simulink model "Quadcopter_ControllerWithNavigation"  (R2023b)
settings: Solver=FixedStepAuto  StartTime=0.0  StopTime=inf  RelTol=1e-3  EnableMultiTasking=on
undefined symbols (not defined in the file): dev, Main, pwm_output0, SampleTime
libraries: slpidlib x10, px4uORBlib x7, simulink x4, px4lib x3, uavalgslib x3, simulink_extras x1, sharedutil x1, sharedtransform x1
(part 2 of 3)

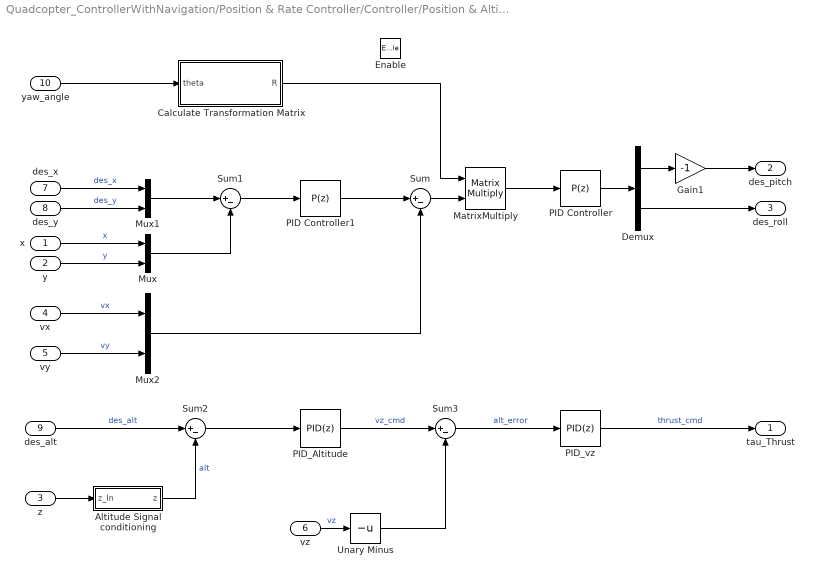
== system Quadcopter_ControllerWithNavigation/Position & Rate Controller/Controller/Position & Altitude controller ==
  x : Inport
  y : Inport  Port=2
  z : Inport  Port=3
  vx : Inport  Port=4
  vy : Inport  Port=5
  vz : Inport  Port=6
  des_x : Inport  Port=7
  des_y : Inport  Port=8
  des_alt : Inport  Port=9
  yaw_angle : Inport  Port=10
  Enable : EnablePort
  Altitude Signal conditioning : Subsystem
  Calculate Transformation Matrix : Subsystem
  Demux : Demux  Outputs=2
  Gain1 : Gain  Gain=-1
  MatrixMultiply : Product  Multiplication=Matrix(*)
  Mux : Mux  Inputs=2
  Mux1 : Mux  Inputs=2
  Mux2 : Mux  Inputs=2
  PID Controller : slpidlib/PID Controller  Controller=P  Form=Parallel  TimeDomain=Discrete-time  UseExternalTs=off  SampleTime=-1  IntegratorMethod=Forward Euler  FilterMethod=Forward Euler  ControllerParametersSource=internal  P=0.3  I=0  UseKiTs=off  D=0  N=20  UseFilter=on  TunerSelectOption=Transfer Function Based (PID Tuner App)  InitialConditionSource=internal  InitialConditionForIntegrator=0  InitialConditionForFilter=0  DifferentiatorICPrevScaledInput=0  ExternalReset=none  TrackingMode=off  Kt=1  LimitOutput=on  SatLimitsSource=internal  UpperSaturationLimit=20*pi/180  LowerSaturationLimit=-20*pi/180  LinearizeAsGain=on  AntiWindupMode=clamping  Kb=1  LimitIntegrator=off  UpperIntegratorSaturationLimit=inf  LowerIntegratorSaturationLimit=-inf  POutMin=[]  POutMax=[]  IOutMin=[]  IOutMax=[]  DOutMin=[]  DOutMax=[]  NOutMin=[]  NOutMax=[]  SumOutMin=[]  SumOutMax=[]  SaturationOutMin=[]  SaturationOutMax=[]  PParamMin=[]  PParamMax=[]  IParamMin=[]  IParamMax=[]  DParamMin=[]  DParamMax=[]  NParamMin=[]  NParamMax=[]  KbParamMin=[]  KbParamMax=[]  KtParamMin=[]  KtParamMax=[]  KbOutMin=[]  KbOutMax=[]  KtOutMin=[]  KtOutMax=[]  IntegratorOutMin=[]  IntegratorOutMax=[]  FilterOutMin=[]  FilterOutMax=[]  SumI1OutMin=[]  SumI1OutMax=[]  SumI2OutMin=[]  SumI2OutMax=[]  SumI3OutMin=[]  SumI3OutMax=[]  SumI4OutMin=[]  SumI4OutMax=[]  SumDOutMin=[]  SumDOutMax=[]  DifferentiatorOutMin=[]  DifferentiatorOutMax=[]  FilterDiffOutCoefMin=[]  FilterDiffOutCoefMax=[]  ReciprocalOutMin=[]  ReciprocalOutMax=[]  SumDenOutMin=[]  SumDenOutMax=[]  SumNumOutMin=[]  SumNumOutMax=[]  DivideOutMin=[]  DivideOutMax=[]  UdiffTsProdOutMin=[]  UdiffTsProdOutMax=[]  NTsProdOutMin=[]  NTsProdOutMax=[]  UintegralTsProdOutMin=[]  UintegralTsProdOutMax=[]  UngainTsProdOutMin=[]  UngainTsProdOutMax=[]  ClampingZeroOutDataTypeStr=Inherit: Inherit via back propagation  ClampingZeroOutMin=[]  ClampingZeroOutMax=[]  FilterDenConstantOutDataTypeStr=Inherit: Inherit via back propagation  FilterDenConstantOutMin=[]  FilterDenConstantOutMax=[]  PCopyOutDataTypeStr=Inherit: Inherit via back propagation  PCopyOutMin=[]  PCopyOutMax=[]  NCopyOutDataTypeStr=Inherit: Inherit via back propagation  NCopyOutMin=[]  NCopyOutMax=[]  IntegratorContinuousStateAttributes=''  IntegratorStateMustResolveToSignalObject=off  IntegratorRTWStateStorageClass=Auto  FilterContinuousStateAttributes=''  FilterStateMustResolveToSignalObject=off  FilterRTWStateStorageClass=Auto  ParallelPVariant=InternalParameters  IdealPVariant=Disabled  IVariant=Disabled  DVariant=Disabled  IntegratorVariant=Disabled  SatVariant=Enabled  AWVariant=Disabled  PCopyVariant=Disabled  TRVariant=Disabled  FdbkBlocksVariant=Forward  IdealPFdbkVariant=Disabled  SatFdbkVariant=Disabled  DerivativeFilterVariant=Disabled  NVariant=Disabled  NCopyVariant=Disabled_SignalSpec  FilterICVariant=Disabled  IntegratorICVariant=Disabled  ExternalResetVariant=Disabled  TRSumVariant=Passthrough  SumFdbkVariant=Disabled  SumVariant=Passthrough_P  TsampFilterVariant=InternalTs  TsampNgainVariant=Passthrough  TsampIntegralVariant=Disabled_SignalSpec  ExternalSaturationOutDataTypeStr=Inherit: Same as second input
  PID Controller1 : slpidlib/PID Controller  Controller=P  Form=Parallel  TimeDomain=Discrete-time  UseExternalTs=off  SampleTime=-1  IntegratorMethod=Forward Euler  FilterMethod=Forward Euler  ControllerParametersSource=internal  P=0.6  I=0  UseKiTs=off  D=0  N=20  UseFilter=on  TunerSelectOption=Transfer Function Based (PID Tuner App)  InitialConditionSource=internal  InitialConditionForIntegrator=0  InitialConditionForFilter=0  DifferentiatorICPrevScaledInput=0  ExternalReset=none  TrackingMode=off  Kt=1  LimitOutput=on  SatLimitsSource=internal  UpperSaturationLimit=4  LowerSaturationLimit=-4  LinearizeAsGain=on  AntiWindupMode=clamping  Kb=1  LimitIntegrator=off  UpperIntegratorSaturationLimit=inf  LowerIntegratorSaturationLimit=-inf  POutMin=[]  POutMax=[]  IOutMin=[]  IOutMax=[]  DOutMin=[]  DOutMax=[]  NOutMin=[]  NOutMax=[]  SumOutMin=[]  SumOutMax=[]  SaturationOutMin=[]  SaturationOutMax=[]  PParamMin=[]  PParamMax=[]  IParamMin=[]  IParamMax=[]  DParamMin=[]  DParamMax=[]  NParamMin=[]  NParamMax=[]  KbParamMin=[]  KbParamMax=[]  KtParamMin=[]  KtParamMax=[]  KbOutMin=[]  KbOutMax=[]  KtOutMin=[]  KtOutMax=[]  IntegratorOutMin=[]  IntegratorOutMax=[]  FilterOutMin=[]  FilterOutMax=[]  SumI1OutMin=[]  SumI1OutMax=[]  SumI2OutMin=[]  SumI2OutMax=[]  SumI3OutMin=[]  SumI3OutMax=[]  SumI4OutMin=[]  SumI4OutMax=[]  SumDOutMin=[]  SumDOutMax=[]  DifferentiatorOutMin=[]  DifferentiatorOutMax=[]  FilterDiffOutCoefMin=[]  FilterDiffOutCoefMax=[]  ReciprocalOutMin=[]  ReciprocalOutMax=[]  SumDenOutMin=[]  SumDenOutMax=[]  SumNumOutMin=[]  SumNumOutMax=[]  DivideOutMin=[]  DivideOutMax=[]  UdiffTsProdOutMin=[]  UdiffTsProdOutMax=[]  NTsProdOutMin=[]  NTsProdOutMax=[]  UintegralTsProdOutMin=[]  UintegralTsProdOutMax=[]  UngainTsProdOutMin=[]  UngainTsProdOutMax=[]  ClampingZeroOutDataTypeStr=Inherit: Inherit via back propagation  ClampingZeroOutMin=[]  ClampingZeroOutMax=[]  FilterDenConstantOutDataTypeStr=Inherit: Inherit via back propagation  FilterDenConstantOutMin=[]  FilterDenConstantOutMax=[]  PCopyOutDataTypeStr=Inherit: Inherit via back propagation  PCopyOutMin=[]  PCopyOutMax=[]  NCopyOutDataTypeStr=Inherit: Inherit via back propagation  NCopyOutMin=[]  NCopyOutMax=[]  IntegratorContinuousStateAttributes=''  IntegratorStateMustResolveToSignalObject=off  IntegratorRTWStateStorageClass=Auto  FilterContinuousStateAttributes=''  FilterStateMustResolveToSignalObject=off  FilterRTWStateStorageClass=Auto  ParallelPVariant=InternalParameters  IdealPVariant=Disabled  IVariant=Disabled  DVariant=Disabled  IntegratorVariant=Disabled  SatVariant=Enabled  AWVariant=Disabled  PCopyVariant=Disabled  TRVariant=Disabled  FdbkBlocksVariant=Forward  IdealPFdbkVariant=Disabled  SatFdbkVariant=Disabled  DerivativeFilterVariant=Disabled  NVariant=Disabled  NCopyVariant=Disabled_SignalSpec  FilterICVariant=Disabled  IntegratorICVariant=Disabled  ExternalResetVariant=Disabled  TRSumVariant=Passthrough  SumFdbkVariant=Disabled  SumVariant=Passthrough_P  TsampFilterVariant=InternalTs  TsampNgainVariant=Passthrough  TsampIntegralVariant=Disabled_SignalSpec  ExternalSaturationOutDataTypeStr=Inherit: Same as second input
  PID_Altitude : slpidlib/PID Controller  Controller=PID  Form=Parallel  TimeDomain=Discrete-time  UseExternalTs=off  SampleTime=-1  IntegratorMethod=Backward Euler  FilterMethod=Forward Euler  ControllerParametersSource=internal  P=1.5  I=0.01  UseKiTs=off  D=0.01  N=10  UseFilter=on  TunerSelectOption=Transfer Function Based (PID Tuner App)  InitialConditionSource=internal  InitialConditionForIntegrator=0  InitialConditionForFilter=0  DifferentiatorICPrevScaledInput=0  ExternalReset=none  TrackingMode=off  Kt=1  LimitOutput=on  SatLimitsSource=internal  UpperSaturationLimit=2  LowerSaturationLimit=-2  LinearizeAsGain=off  AntiWindupMode=clamping  Kb=1  LimitIntegrator=off  UpperIntegratorSaturationLimit=inf  LowerIntegratorSaturationLimit=-inf  POutMin=[]  POutMax=[]  IOutMin=[]  IOutMax=[]  DOutMin=[]  DOutMax=[]  NOutMin=[]  NOutMax=[]  SumOutMin=[]  SumOutMax=[]  SaturationOutMin=[]  SaturationOutMax=[]  PParamMin=[]  PParamMax=[]  IParamMin=[]  IParamMax=[]  DParamMin=[]  DParamMax=[]  NParamMin=[]  NParamMax=[]  KbParamMin=[]  KbParamMax=[]  KtParamMin=[]  KtParamMax=[]  KbOutMin=[]  KbOutMax=[]  KtOutMin=[]  KtOutMax=[]  IntegratorOutMin=[]  IntegratorOutMax=[]  FilterOutMin=[]  FilterOutMax=[]  SumI1OutMin=[]  SumI1OutMax=[]  SumI2OutMin=[]  SumI2OutMax=[]  SumI3OutMin=[]  SumI3OutMax=[]  SumI4OutMin=[]  SumI4OutMax=[]  SumDOutMin=[]  SumDOutMax=[]  DifferentiatorOutMin=[]  DifferentiatorOutMax=[]  FilterDiffOutCoefMin=[]  FilterDiffOutCoefMax=[]  ReciprocalOutMin=[]  ReciprocalOutMax=[]  SumDenOutMin=[]  SumDenOutMax=[]  SumNumOutMin=[]  SumNumOutMax=[]  DivideOutMin=[]  DivideOutMax=[]  UdiffTsProdOutMin=[]  UdiffTsProdOutMax=[]  NTsProdOutMin=[]  NTsProdOutMax=[]  UintegralTsProdOutMin=[]  UintegralTsProdOutMax=[]  UngainTsProdOutMin=[]  UngainTsProdOutMax=[]  ClampingZeroOutDataTypeStr=Inherit: Inherit via back propagation  ClampingZeroOutMin=[]  ClampingZeroOutMax=[]  FilterDenConstantOutDataTypeStr=Inherit: Inherit via back propagation  FilterDenConstantOutMin=[]  FilterDenConstantOutMax=[]  PCopyOutDataTypeStr=Inherit: Inherit via back propagation  PCopyOutMin=[]  PCopyOutMax=[]  NCopyOutDataTypeStr=Inherit: Inherit via back propagation  NCopyOutMin=[]  NCopyOutMax=[]  IntegratorContinuousStateAttributes=''  IntegratorStateMustResolveToSignalObject=off  IntegratorRTWStateStorageClass=Auto  FilterContinuousStateAttributes=''  FilterStateMustResolveToSignalObject=off  FilterRTWStateStorageClass=Auto  ParallelPVariant=InternalParameters  IdealPVariant=Disabled  IVariant=InternalParameters  DVariant=InternalParameters  IntegratorVariant=Discrete  SatVariant=Enabled  AWVariant=DiscClampingParallel  PCopyVariant=Disabled  TRVariant=Disabled  FdbkBlocksVariant=Feedback  IdealPFdbkVariant=Passthrough  SatFdbkVariant=Passthrough  DerivativeFilterVariant=ForwardEulerFilter  NVariant=InternalParameters  NCopyVariant=Disabled  FilterICVariant=InternalICsFilter  IntegratorICVariant=InternalICs  ExternalResetVariant=Disabled  TRSumVariant=Passthrough  SumFdbkVariant=Enabled  SumVariant=Sum_PID  TsampFilterVariant=InternalTs  TsampNgainVariant=Passthrough  TsampIntegralVariant=Disabled_SignalSpec  ExternalSaturationOutDataTypeStr=Inherit: Same as second input
  PID_vz : slpidlib/PID Controller  Controller=PID  Form=Parallel  TimeDomain=Discrete-time  UseExternalTs=off  SampleTime=-1  IntegratorMethod=Backward Euler  FilterMethod=Forward Euler  ControllerParametersSource=internal  P=0.5  I=0.1  UseKiTs=off  D=0.05  N=10  UseFilter=on  TunerSelectOption=Transfer Function Based (PID Tuner App)  InitialConditionSource=internal  InitialConditionForIntegrator=0  InitialConditionForFilter=0  DifferentiatorICPrevScaledInput=0  ExternalReset=none  TrackingMode=off  Kt=1  LimitOutput=on  SatLimitsSource=internal  UpperSaturationLimit=1  LowerSaturationLimit=0  LinearizeAsGain=off  AntiWindupMode=clamping  Kb=1  LimitIntegrator=off  UpperIntegratorSaturationLimit=inf  LowerIntegratorSaturationLimit=-inf  POutMin=[]  POutMax=[]  IOutMin=[]  IOutMax=[]  DOutMin=[]  DOutMax=[]  NOutMin=[]  NOutMax=[]  SumOutMin=[]  SumOutMax=[]  SaturationOutMin=[]  SaturationOutMax=[]  PParamMin=[]  PParamMax=[]  IParamMin=[]  IParamMax=[]  DParamMin=[]  DParamMax=[]  NParamMin=[]  NParamMax=[]  KbParamMin=[]  KbParamMax=[]  KtParamMin=[]  KtParamMax=[]  KbOutMin=[]  KbOutMax=[]  KtOutMin=[]  KtOutMax=[]  IntegratorOutMin=[]  IntegratorOutMax=[]  FilterOutMin=[]  FilterOutMax=[]  SumI1OutMin=[]  SumI1OutMax=[]  SumI2OutMin=[]  SumI2OutMax=[]  SumI3OutMin=[]  SumI3OutMax=[]  SumI4OutMin=[]  SumI4OutMax=[]  SumDOutMin=[]  SumDOutMax=[]  DifferentiatorOutMin=[]  DifferentiatorOutMax=[]  FilterDiffOutCoefMin=[]  FilterDiffOutCoefMax=[]  ReciprocalOutMin=[]  ReciprocalOutMax=[]  SumDenOutMin=[]  SumDenOutMax=[]  SumNumOutMin=[]  SumNumOutMax=[]  DivideOutMin=[]  DivideOutMax=[]  UdiffTsProdOutMin=[]  UdiffTsProdOutMax=[]  NTsProdOutMin=[]  NTsProdOutMax=[]  UintegralTsProdOutMin=[]  UintegralTsProdOutMax=[]  UngainTsProdOutMin=[]  UngainTsProdOutMax=[]  ClampingZeroOutDataTypeStr=Inherit: Inherit via back propagation  ClampingZeroOutMin=[]  ClampingZeroOutMax=[]  FilterDenConstantOutDataTypeStr=Inherit: Inherit via back propagation  FilterDenConstantOutMin=[]  FilterDenConstantOutMax=[]  PCopyOutDataTypeStr=Inherit: Inherit via back propagation  PCopyOutMin=[]  PCopyOutMax=[]  NCopyOutDataTypeStr=Inherit: Inherit via back propagation  NCopyOutMin=[]  NCopyOutMax=[]  IntegratorContinuousStateAttributes=''  IntegratorStateMustResolveToSignalObject=off  IntegratorRTWStateStorageClass=Auto  FilterContinuousStateAttributes=''  FilterStateMustResolveToSignalObject=off  FilterRTWStateStorageClass=Auto  ParallelPVariant=InternalParameters  IdealPVariant=Disabled  IVariant=InternalParameters  DVariant=InternalParameters  IntegratorVariant=Discrete  SatVariant=Enabled  AWVariant=DiscClampingParallel  PCopyVariant=Disabled  TRVariant=Disabled  FdbkBlocksVariant=Feedback  IdealPFdbkVariant=Passthrough  SatFdbkVariant=Passthrough  DerivativeFilterVariant=ForwardEulerFilter  NVariant=InternalParameters  NCopyVariant=Disabled  FilterICVariant=InternalICsFilter  IntegratorICVariant=InternalICs  ExternalResetVariant=Disabled  TRSumVariant=Passthrough  SumFdbkVariant=Enabled  SumVariant=Sum_PID  TsampFilterVariant=InternalTs  TsampNgainVariant=Passthrough  TsampIntegralVariant=Disabled_SignalSpec  ExternalSaturationOutDataTypeStr=Inherit: Same as second input
  Sum{,1..3} (4 alike) : Sum  Inputs=|+-
  Unary Minus : UnaryMinus
  tau_Thrust : Outport
  des_pitch : Outport  Port=2
  des_roll : Outport  Port=3
  wires:
  des_alt/1 -> Sum2/1  "des_alt"
  Calculate Transformation Matrix/1(R) -> MatrixMultiply/1
  yaw_angle/1 -> Calculate Transformation Matrix/1(theta)
  Altitude Signal conditioning/1(z) -> Sum2/2  "alt"
  PID_Altitude/1 -> Sum3/1  "vz_cmd"
  vz/1 -> Unary Minus/1  "vz"
  PID_vz/1 -> tau_Thrust/1  "thrust_cmd"
  vx/1 -> Mux2/1  "vx"
  vy/1 -> Mux2/2  "vy"
  Sum2/1 -> PID_Altitude/1
  z/1 -> Altitude Signal conditioning/1(z_In)
  PID Controller/1 -> Demux/1
  Demux/1 -> Gain1/1
  x/1 -> Mux/1  "x"
  y/1 -> Mux/2  "y"
  Mux2/1 -> Sum/2
  Gain1/1 -> des_pitch/1
  Demux/2 -> des_roll/1
  Sum/1 -> MatrixMultiply/2
  Mux/1 -> Sum1/2
  Sum1/1 -> PID Controller1/1
  Unary Minus/1 -> Sum3/2
  Sum3/1 -> PID_vz/1  "alt_error"
  des_x/1 -> Mux1/1  "des_x"
  des_y/1 -> Mux1/2  "des_y"
  MatrixMultiply/1 -> PID Controller/1
  PID Controller1/1 -> Sum/1
  Mux1/1 -> Sum1/1

== system Quadcopter_ControllerWithNavigation/Position & Rate Controller/Controller/Quaternion Validity Check ==
  In1 : Inport
  Constant : Constant  Value=[1 0 0 0]  SampleTime=-1
  Quaternion Norm : sharedutil/Quaternion Norm  aMode=aMode
  Switch : Switch  Criteria=u2 > Threshold  SaturateOnIntegerOverflow=off  InputSameDT=off
  Valid quat : Outport
  wires:
  In1/1 -> Quaternion Norm/1, Switch/1
  Quaternion Norm/1 -> Switch/2
  Switch/1 -> Valid quat/1
  Constant/1 -> Switch/3

== system Quadcopter_ControllerWithNavigation/Navigation/Quadcopter Navigation Algorithm/Manual Waypoints/Subsystem ==
  curr_xyzYaw : Inport
  Lookahead Point : Inport  Port=2
  Add : Sum  Inputs=+-
  Constant : Constant  Value=-1  OutDataTypeStr=Inherit: Inherit via back propagation
  Constant2 : Constant  Value=0  OutDataTypeStr=Inherit: Inherit via back propagation
  Gain : Gain
  Mux : Mux  Inputs=2
  Saturation Dynamic1 : simulink/Discontinuities/Saturation Dynamic  OutMin=0  OutMax=[]  OutDataTypeStr=Inherit: Same as second input  OutDataType=fixdt(1, 16)  OutScaling=2^-10  DoSatur=off
  Selector : Selector  InputPortWidth=4  IndexOptions=Index vector (dialog)  Indices=[3]  OutputSizes=1
  Selector1 : Selector  InputPortWidth=3  IndexOptions=Index vector (dialog)  Indices=[1 2]  OutputSizes=1
  des_landing_pos : Outport
  wires:
  Gain/1 -> Add/1
  Constant/1 -> Add/2
  Mux/1 -> des_landing_pos/1
  curr_xyzYaw/1 -> Selector/1
  Selector/1 -> Gain/1  "curr_z"
  Lookahead Point/1 -> Selector1/1
  Selector1/1 -> Mux/1  "Lookahead Point xy"
  Constant2/1 -> Saturation Dynamic1/1
  Add/1 -> Saturation Dynamic1/2, Saturation Dynamic1/3
  Saturation Dynamic1/1 -> Mux/2

== system Quadcopter_ControllerWithNavigation/Navigation/Quadcopter Navigation Algorithm/Path Correction from Onboard Computer/Define WP Yaw Values  ==
  position setpoint : Inport
  Trajectory Waypoint : Inport  Port=2
  Bus Selector : BusSelector  OutputSignals=waypoints
  Bus Selector1 : BusSelector  OutputSignals=yaw
  Bus Selector2 : BusSelector  OutputSignals=previous.yaw,next.yaw
  Data Type Conversion : DataTypeConversion  OutDataTypeStr=double  SaturateOnIntegerOverflow=off  RndMeth=Floor
  Data Type Conversion1 : DataTypeConversion  OutDataTypeStr=double  SaturateOnIntegerOverflow=off  RndMeth=Floor
  Data Type Conversion2 : DataTypeConversion  OutDataTypeStr=double  SaturateOnIntegerOverflow=off  RndMeth=Floor
  Selector : Selector  InputPortWidth=5  IndexOptions=Index vector (dialog)  Indices=1  OutputSizes=1
  Previous WP Yaw : Outport
  Current WP Yaw : Outport  Port=2
  Next WP Yaw : Outport  Port=3
  wires:
  Selector/1 -> Bus Selector1/1
  Bus Selector1/1 -> Data Type Conversion2/1  "<yaw>"
  position setpoint/1 -> Bus Selector2/1
  Bus Selector2/1 -> Data Type Conversion/1  "<yaw>"
  Bus Selector2/2 -> Data Type Conversion1/1  "<yaw>"
  Trajectory Waypoint/1 -> Bus Selector/1
  Bus Selector/1 -> Selector/1  "<waypoints>"
  Data Type Conversion/1 -> Previous WP Yaw/1
  Data Type Conversion1/1 -> Next WP Yaw/1
  Data Type Conversion2/1 -> Current WP Yaw/1

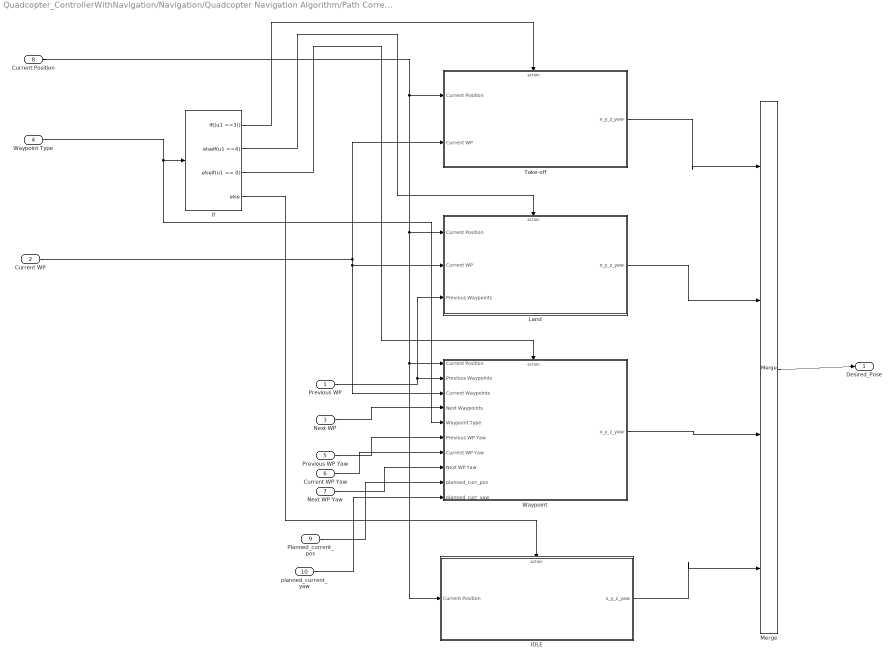
== system Quadcopter_ControllerWithNavigation/Navigation/Quadcopter Navigation Algorithm/Path Correction from Onboard Computer/Guidance Subsystem ==
  Previous WP : Inport
  Current WP : Inport  Port=2
  Next WP : Inport  Port=3
  Waypoint Type : Inport  Port=4
  Previous WP Yaw : Inport  Port=5
  Current WP Yaw : Inport  Port=6
  Next WP Yaw : Inport  Port=7
  Current Position : Inport  Port=8
  Planned_current_pos : Inport  Port=9
  planned_current_yaw : Inport  Port=10
  IDLE : Subsystem  TreatAsAtomicUnit=on
  If : If  IfExpression=(u1 ==3)  ElseIfExpressions=u1 ==4, u1 == 0
  Land : Subsystem  TreatAsAtomicUnit=on
  Merge : Merge  Inputs=4
  Take-off : Subsystem  TreatAsAtomicUnit=on
  Waypoint : Subsystem  TreatAsAtomicUnit=on
  Desired_Pose : Outport
  wires:
  Previous WP/1 -> Land/3(Previous Waypoints), Waypoint/2(Previous Waypoints)
  Current WP/1 -> Land/2(Current WP), Waypoint/3(Current Waypoints), Take-off/2(Current WP)
  Merge/1 -> Desired_Pose/1
  Next WP/1 -> Waypoint/4(Next Waypoints)
  Current Position/1 -> Land/1(Current Position), IDLE/1(Current Position), Waypoint/1(Current Position), Take-off/1(Current Position)
  Waypoint Type/1 -> If/1, Waypoint/5(Waypoint Type)
  If/1 -> Take-off/Action
  Take-off/1(x_y_z_yaw) -> Merge/1
  If/2 -> Land/Action
  Land/1(x_y_z_yaw) -> Merge/2
  Waypoint/1(x_y_z_yaw) -> Merge/3
  Previous WP Yaw/1 -> Waypoint/6(Previous WP Yaw)
  Current WP Yaw/1 -> Waypoint/7(Current WP Yaw)
  Next WP Yaw/1 -> Waypoint/8(Next WP Yaw)
  If/3 -> Waypoint/Action
  IDLE/1(x_y_z_yaw) -> Merge/4
  If/4 -> IDLE/Action
  Planned_current_pos/1 -> Waypoint/9(planned_curr_pos)
  planned_current_yaw/1 -> Waypoint/10(planned_curr_yaw)

== system Quadcopter_ControllerWithNavigation/Navigation/Quadcopter Navigation Algorithm/Path Correction from Onboard Computer/NaN Check ==
  In1 : Inport
  IsNaN : RelationalOperator  Operator=isNaN  OutDataTypeStr=boolean  RndMeth=Simplest  InputSameDT=off
  Switch : Switch  Criteria=u2 > Threshold  SaturateOnIntegerOverflow=off  InputSameDT=off
  previous safe value : Subsystem
  Out1 : Outport
  wires:
  IsNaN/1 -> Switch/2
  previous safe value/1(Out1) -> Switch/1
  Switch/1 -> Out1/1
  In1/1 -> IsNaN/1, Switch/3, previous safe value/1(In1)

== system Quadcopter_ControllerWithNavigation/Navigation/Quadcopter Navigation Algorithm/Path Correction from Onboard Computer/NaN Check1 ==
  In1 : Inport
  IsNaN : RelationalOperator  Operator=isNaN  OutDataTypeStr=boolean  RndMeth=Simplest  InputSameDT=off
  Switch : Switch  Criteria=u2 > Threshold  SaturateOnIntegerOverflow=off  InputSameDT=off
  previous safe value : Subsystem
  Out1 : Outport
  wires:
  In1/1 -> previous safe value/1(In1), Switch/3, IsNaN/1
  Switch/1 -> Out1/1
  previous safe value/1(Out1) -> Switch/1
  IsNaN/1 -> Switch/2

== system Quadcopter_ControllerWithNavigation/Navigation/Quadcopter Navigation Algorithm/Path Correction from Onboard Computer/NaN Check2 ==
  In1 : Inport
  IsNaN : RelationalOperator  Operator=isNaN  OutDataTypeStr=boolean  RndMeth=Simplest  InputSameDT=off
  Switch : Switch  Criteria=u2 > Threshold  SaturateOnIntegerOverflow=off  InputSameDT=off
  previous safe value : Subsystem
  Out1 : Outport
  wires:
  IsNaN/1 -> Switch/2
  previous safe value/1(Out1) -> Switch/1
  Switch/1 -> Out1/1
  In1/1 -> IsNaN/1, Switch/3, previous safe value/1(In1)

== system Quadcopter_ControllerWithNavigation/Navigation/Quadcopter Navigation Algorithm/Path Correction from Onboard Computer/NaN Check3 ==
  In1 : Inport
  IsNaN : RelationalOperator  Operator=isNaN  OutDataTypeStr=boolean  RndMeth=Simplest  InputSameDT=off
  Switch : Switch  Criteria=u2 > Threshold  SaturateOnIntegerOverflow=off  InputSameDT=off
  previous safe value : Subsystem
  Out1 : Outport
  wires:
  In1/1 -> previous safe value/1(In1), Switch/3, IsNaN/1
  Switch/1 -> Out1/1
  previous safe value/1(Out1) -> Switch/1
  IsNaN/1 -> Switch/2

== system Quadcopter_ControllerWithNavigation/Navigation/Quadcopter Navigation Algorithm/Path Correction from Onboard Computer/NaN Check4 ==
  In1 : Inport
  IsNaN : RelationalOperator  Operator=isNaN  OutDataTypeStr=boolean  RndMeth=Simplest  InputSameDT=off
  Switch : Switch  Criteria=u2 > Threshold  SaturateOnIntegerOverflow=off  InputSameDT=off
  previous safe value : Subsystem
  Out1 : Outport
  wires:
  IsNaN/1 -> Switch/2
  previous safe value/1(Out1) -> Switch/1
  Switch/1 -> Out1/1
  In1/1 -> IsNaN/1, Switch/3, previous safe value/1(In1)

== system Quadcopter_ControllerWithNavigation/Navigation/Quadcopter Navigation Algorithm/Path Correction from Onboard Computer/NaN Check5 ==
  In1 : Inport
  IsNaN : RelationalOperator  Operator=isNaN  OutDataTypeStr=boolean  RndMeth=Simplest  InputSameDT=off
  Switch : Switch  Criteria=u2 > Threshold  SaturateOnIntegerOverflow=off  InputSameDT=off
  previous safe value : Subsystem
  Out1 : Outport
  wires:
  In1/1 -> previous safe value/1(In1), Switch/3, IsNaN/1
  Switch/1 -> Out1/1
  previous safe value/1(Out1) -> Switch/1
  IsNaN/1 -> Switch/2

== system Quadcopter_ControllerWithNavigation/Navigation/Quadcopter Navigation Algorithm/Read waypoint from QGroundControl Mission/Guidance Subsystem ==
  Previous WP : Inport
  Current WP : Inport  Port=2
  Next WP : Inport  Port=3
  Waypoint Type : Inport  Port=4
  Current Position : Inport  Port=5
  IDLE : Subsystem  TreatAsAtomicUnit=on
  If : If  IfExpression=(u1 ==3)  ElseIfExpressions=u1 ==4, u1==0
  Land : Subsystem  TreatAsAtomicUnit=on
  Merge : Merge  Inputs=4
  Take-off : Subsystem  TreatAsAtomicUnit=on
  Waypoint : Subsystem  TreatAsAtomicUnit=on
  Desired_Pose : Outport
  wires:
  Previous WP/1 -> Land/3(Previous Waypoints), Waypoint/2(Previous Waypoints)
  Current WP/1 -> Take-off/2(Current WP), Land/2(Current WP), Waypoint/3(Current Waypoints)
  Merge/1 -> Desired_Pose/1
  Next WP/1 -> Waypoint/4(Next Waypoints)
  Current Position/1 -> Take-off/1(Current Position), Land/1(Current Position), IDLE/1(Current Position), Waypoint/1(Current Position)
  Waypoint Type/1 -> Waypoint/5(Waypoint Type), If/1
  If/1 -> Take-off/Action
  If/4 -> IDLE/Action
  Take-off/1(x_y_z_yaw) -> Merge/1
  If/2 -> Land/Action
  Land/1(x_y_z_yaw) -> Merge/2
  Waypoint/1(x_y_z_yaw) -> Merge/3
  IDLE/1(x_y_z_yaw) -> Merge/4
  If/3 -> Waypoint/Action

== system Quadcopter_ControllerWithNavigation/Position & Rate Controller/Controller/Attitude controller/Calculate minimum Turn ==
  In1 : Inport
  Abs : Abs  SaturateOnIntegerOverflow=off
  Add : Sum
  Constant : Constant  Value=2*pi  SampleTime=-1
  Subtract : Sum  Inputs=+-
  Switch : Switch  Criteria=u2 > Threshold  Threshold=pi  SaturateOnIntegerOverflow=off  InputSameDT=off
  Switch1 : Switch  Criteria=u2 > Threshold  SaturateOnIntegerOverflow=off  InputSameDT=off
  Out1 : Outport
  wires:
  Switch/1 -> Out1/1
  Abs/1 -> Switch/2
  Constant/1 -> Subtract/2, Add/1
  Subtract/1 -> Switch1/1
  Add/1 -> Switch1/3
  In1/1 -> Subtract/1, Switch/3, Abs/1, Switch1/2, Add/2
  Switch1/1 -> Switch/1

== system Quadcopter_ControllerWithNavigation/Position & Rate Controller/Controller/Position & Altitude controller/Altitude Signal conditioning ==
  z_In : Inport
  Constant : Constant  Value=0
  Gain1 : Gain  Gain=-1
  Saturation Dynamic : simulink/Discontinuities/Saturation Dynamic  OutMin=[]  OutMax=[]  OutDataTypeStr=Inherit: Same as second input  OutDataType=fixdt(1, 16)  OutScaling=2^-10  DoSatur=off
  z : Outport
  wires:
  z_In/1 -> Gain1/1
  Gain1/1 -> Saturation Dynamic/1, Saturation Dynamic/2
  Constant/1 -> Saturation Dynamic/3
  Saturation Dynamic/1 -> z/1  "alt"

== system Quadcopter_ControllerWithNavigation/Position & Rate Controller/Controller/Position & Altitude controller/Calculate Transformation Matrix ==
  theta : Inport
  Gain : Gain  Gain=-1
  Matrix Concatenate : Concatenate  Mode=Multidimensional array
  Mux : Mux  Inputs=2
  Mux1 : Mux  Inputs=2
  Reshape : Reshape  OutputDimensionality=Row vector (2-D)
  Reshape1 : Reshape  OutputDimensionality=Row vector (2-D)
  SinCos : Trigonometry  Operator=sincos
  Transpose : Math  Operator=transpose
  R : Outport
  wires:
  theta/1 -> SinCos/1
  SinCos/2 -> Mux1/2, Mux/1
  SinCos/1 -> Gain/1, Mux1/1
  Gain/1 -> Mux/2
  Mux/1 -> Reshape/1
  Mux1/1 -> Reshape1/1
  Matrix Concatenate/1 -> Transpose/1
  Transpose/1 -> R/1
  Reshape/1 -> Matrix Concatenate/1
  Reshape1/1 -> Matrix Concatenate/2

== system Quadcopter_ControllerWithNavigation/Navigation/Quadcopter Navigation Algorithm/Path Correction from Onboard Computer/Guidance Subsystem/IDLE ==
  Current Position : Inport
  Action Port : ActionPort  InitializeStates=reset
  Maintain Current Yaw during IDLE : Subsystem
  Mux : Mux  Inputs=2
  Reshape1 : Reshape  OutputDimensionality=Row vector (2-D)
  Selector : Selector  InputPortWidth=4  IndexOptions=Index vector (dialog)  Indices=[4]  OutputSizes=1
  Selector1 : Selector  InputPortWidth=4  IndexOptions=Index vector (dialog)  Indices=[1 2 3]  OutputSizes=1
  x_y_z_yaw : Outport
  wires:
  Maintain Current Yaw during IDLE/1(yaw_Out) -> Mux/2
  Current Position/1 -> Selector/1, Selector1/1
  Selector/1 -> Maintain Current Yaw during IDLE/1(yaw_In)
  Selector1/1 -> Mux/1
  Mux/1 -> Reshape1/1
  Reshape1/1 -> x_y_z_yaw/1

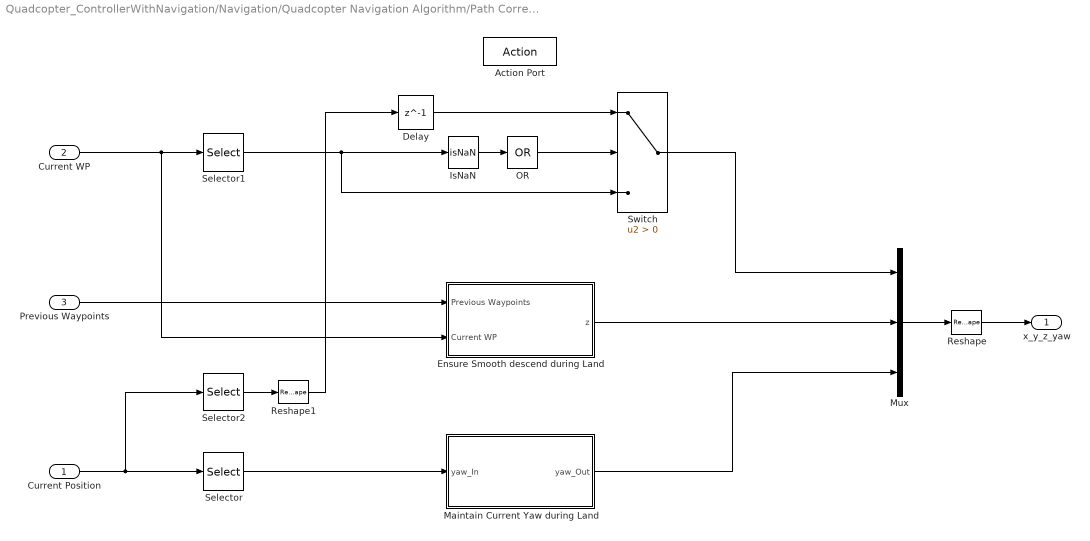
== system Quadcopter_ControllerWithNavigation/Navigation/Quadcopter Navigation Algorithm/Path Correction from Onboard Computer/Guidance Subsystem/Land ==
  Current Position : Inport
  Current WP : Inport  Port=2
  Previous Waypoints : Inport  Port=3
  Action Port : ActionPort  InitializeStates=reset
  Delay : Delay  DelayLength=1
  Ensure Smooth descend during Land : Subsystem
  IsNaN : RelationalOperator  Operator=isNaN  OutDataTypeStr=boolean  RndMeth=Simplest  InputSameDT=off
  Maintain Current Yaw during Land : Subsystem
  Mux : Mux  Inputs=3
  OR : Logic  Operator=OR  Inputs=1  IconShape=distinctive  AllPortsSameDT=off  OutDataTypeStr=boolean
  Reshape : Reshape  OutputDimensionality=Row vector (2-D)
  Reshape1 : Reshape  OutputDimensionality=Row vector (2-D)
  Selector : Selector  InputPortWidth=4  IndexOptions=Index vector (dialog)  Indices=[4]  OutputSizes=1
  Selector1 : Selector  InputPortWidth=3  IndexOptions=Index vector (dialog)  Indices=[1 2]  OutputSizes=1
  Selector2 : Selector  InputPortWidth=4  IndexOptions=Index vector (dialog)  Indices=[1 2]  OutputSizes=1
  Switch : Switch  Criteria=u2 > Threshold  SaturateOnIntegerOverflow=off  InputSameDT=off
  x_y_z_yaw : Outport
  wires:
  Maintain Current Yaw during Land/1(yaw_Out) -> Mux/3
  Selector1/1 -> Switch/3, IsNaN/1
  Ensure Smooth descend during Land/1(z) -> Mux/2
  Previous Waypoints/1 -> Ensure Smooth descend during Land/1(Previous Waypoints)
  Selector/1 -> Maintain Current Yaw during Land/1(yaw_In)
  Switch/1 -> Mux/1
  Current WP/1 -> Ensure Smooth descend during Land/2(Current WP), Selector1/1
  IsNaN/1 -> OR/1
  Selector2/1 -> Reshape1/1
  Reshape1/1 -> Delay/1
  OR/1 -> Switch/2
  Mux/1 -> Reshape/1
  Current Position/1 -> Selector2/1, Selector/1
  Reshape/1 -> x_y_z_yaw/1
  Delay/1 -> Switch/1

== system Quadcopter_ControllerWithNavigation/Navigation/Quadcopter Navigation Algorithm/Path Correction from Onboard Computer/Guidance Subsystem/Take-off ==
  Current Position : Inport
  Current WP : Inport  Port=2
  Action Port : ActionPort  InitializeStates=reset
  Demux : Demux
  Demux1 : Demux  Outputs=3
  Ensure smooth ascend during Takeoff : Subsystem
  Maintain Current Yaw during TakeOff : Subsystem
  Mux : Mux
  Reshape : Reshape  OutputDimensionality=Row vector (2-D)
  Terminator1 : Terminator
  Terminator2 : Terminator
  Terminator3 : Terminator
  x_y_z_yaw : Outport
  wires:
  Current Position/1 -> Demux/1
  Mux/1 -> Reshape/1
  Current WP/1 -> Demux1/1
  Demux/3 -> Terminator3/1
  Demux/1 -> Terminator1/1
  Demux/2 -> Terminator2/1
  Demux1/1 -> Mux/1
  Demux1/2 -> Mux/2
  Reshape/1 -> x_y_z_yaw/1
  Demux/4 -> Maintain Current Yaw during TakeOff/1(yaw_In)
  Maintain Current Yaw during TakeOff/1(yaw_Out) -> Mux/4
  Ensure smooth ascend during Takeoff/1(Out1) -> Mux/3
  Demux1/3 -> Ensure smooth ascend during Takeoff/1(In1)

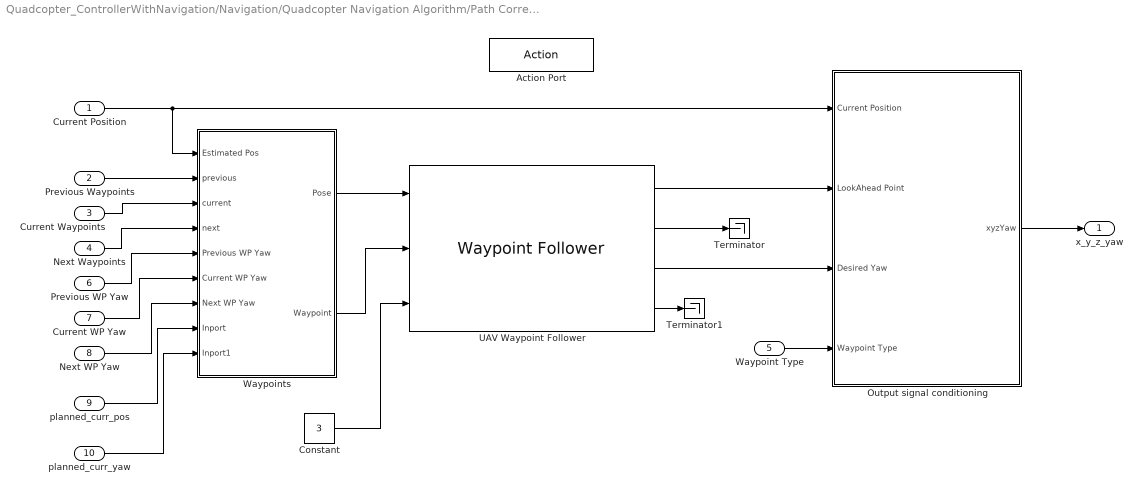
== system Quadcopter_ControllerWithNavigation/Navigation/Quadcopter Navigation Algorithm/Path Correction from Onboard Computer/Guidance Subsystem/Waypoint ==
  Current Position : Inport
  Previous Waypoints : Inport  Port=2
  Current Waypoints : Inport  Port=3
  Next Waypoints : Inport  Port=4
  Waypoint Type : Inport  Port=5
  Previous WP Yaw : Inport  Port=6
  Current WP Yaw : Inport  Port=7
  Next WP Yaw : Inport  Port=8
  planned_curr_pos : Inport  Port=9
  planned_curr_yaw : Inport  Port=10
  Action Port : ActionPort  InitializeStates=reset
  Constant : Constant  Value=3
  Output signal conditioning : Subsystem
  Terminator : Terminator
  Terminator1 : Terminator
  UAV Waypoint Follower : uavalgslib/Waypoint Follower  UAVType=multirotor  StartFrom=first  TransitionRadiusSource=internal  TransitionRadius=2  MinLookaheadDistance=0.3  YawInput=on  ShowCrossTrackErrorOutput=off  ShowStatusOutput=off  SimulateUsing=Code generation
  Waypoints : Subsystem
  x_y_z_yaw : Outport
  wires:
  UAV Waypoint Follower/2 -> Terminator/1
  UAV Waypoint Follower/4 -> Terminator1/1
  Waypoints/2(Waypoint) -> UAV Waypoint Follower/2
  Previous Waypoints/1 -> Waypoints/2(previous)
  Current Waypoints/1 -> Waypoints/3(current)
  Output signal conditioning/1(xyzYaw) -> x_y_z_yaw/1
  Next Waypoints/1 -> Waypoints/4(next)
  UAV Waypoint Follower/3 -> Output signal conditioning/3(Desired Yaw)
  Waypoint Type/1 -> Output signal conditioning/4(Waypoint Type)
  Current Position/1 -> Waypoints/1(Estimated Pos), Output signal conditioning/1(Current Position)
  Previous WP Yaw/1 -> Waypoints/5(Previous WP Yaw)
  Current WP Yaw/1 -> Waypoints/6(Current WP Yaw)
  Next WP Yaw/1 -> Waypoints/7(Next WP Yaw)
  UAV Waypoint Follower/1 -> Output signal conditioning/2(LookAhead Point)
  Waypoints/1(Pose) -> UAV Waypoint Follower/1
  Constant/1 -> UAV Waypoint Follower/3
  planned_curr_pos/1 -> Waypoints/8(Inport)
  planned_curr_yaw/1 -> Waypoints/9(Inport1)

== system Quadcopter_ControllerWithNavigation/Navigation/Quadcopter Navigation Algorithm/Path Correction from Onboard Computer/NaN Check/previous safe value ==
  In1 : Inport
  Delay : Delay  DelayLength=1
  IsNaN1 : RelationalOperator  Operator=isNaN  OutDataTypeStr=boolean  RndMeth=Simplest  InputSameDT=off
  Switch1 : Switch  Criteria=u2 > Threshold  SaturateOnIntegerOverflow=off  InputSameDT=off
  Out1 : Outport
  wires:
  IsNaN1/1 -> Switch1/2
  Delay/1 -> Switch1/1
  Switch1/1 -> Delay/1, Out1/1
  In1/1 -> IsNaN1/1, Switch1/3

== system Quadcopter_ControllerWithNavigation/Navigation/Quadcopter Navigation Algorithm/Path Correction from Onboard Computer/NaN Check1/previous safe value ==
  In1 : Inport
  Delay : Delay  DelayLength=1
  IsNaN1 : RelationalOperator  Operator=isNaN  OutDataTypeStr=boolean  RndMeth=Simplest  InputSameDT=off
  Switch1 : Switch  Criteria=u2 > Threshold  SaturateOnIntegerOverflow=off  InputSameDT=off
  Out1 : Outport
  wires:
  In1/1 -> Switch1/3, IsNaN1/1
  Switch1/1 -> Out1/1, Delay/1
  Delay/1 -> Switch1/1
  IsNaN1/1 -> Switch1/2

== system Quadcopter_ControllerWithNavigation/Navigation/Quadcopter Navigation Algorithm/Path Correction from Onboard Computer/NaN Check2/previous safe value ==
  In1 : Inport
  Delay : Delay  DelayLength=1
  IsNaN1 : RelationalOperator  Operator=isNaN  OutDataTypeStr=boolean  RndMeth=Simplest  InputSameDT=off
  Switch1 : Switch  Criteria=u2 > Threshold  SaturateOnIntegerOverflow=off  InputSameDT=off
  Out1 : Outport
  wires:
  IsNaN1/1 -> Switch1/2
  Delay/1 -> Switch1/1
  Switch1/1 -> Delay/1, Out1/1
  In1/1 -> IsNaN1/1, Switch1/3

== system Quadcopter_ControllerWithNavigation/Navigation/Quadcopter Navigation Algorithm/Path Correction from Onboard Computer/NaN Check3/previous safe value ==
  In1 : Inport
  Delay : Delay  DelayLength=1
  IsNaN1 : RelationalOperator  Operator=isNaN  OutDataTypeStr=boolean  RndMeth=Simplest  InputSameDT=off
  Switch1 : Switch  Criteria=u2 > Threshold  SaturateOnIntegerOverflow=off  InputSameDT=off
  Out1 : Outport
  wires:
  In1/1 -> Switch1/3, IsNaN1/1
  Switch1/1 -> Out1/1, Delay/1
  Delay/1 -> Switch1/1
  IsNaN1/1 -> Switch1/2

== system Quadcopter_ControllerWithNavigation/Navigation/Quadcopter Navigation Algorithm/Path Correction from Onboard Computer/NaN Check4/previous safe value ==
  In1 : Inport
  Delay : Delay  DelayLength=1
  IsNaN1 : RelationalOperator  Operator=isNaN  OutDataTypeStr=boolean  RndMeth=Simplest  InputSameDT=off
  Switch1 : Switch  Criteria=u2 > Threshold  SaturateOnIntegerOverflow=off  InputSameDT=off
  Out1 : Outport
  wires:
  IsNaN1/1 -> Switch1/2
  Delay/1 -> Switch1/1
  Switch1/1 -> Delay/1, Out1/1
  In1/1 -> IsNaN1/1, Switch1/3

== system Quadcopter_ControllerWithNavigation/Navigation/Quadcopter Navigation Algorithm/Path Correction from Onboard Computer/NaN Check5/previous safe value ==
  In1 : Inport
  Delay : Delay  DelayLength=1
  IsNaN1 : RelationalOperator  Operator=isNaN  OutDataTypeStr=boolean  RndMeth=Simplest  InputSameDT=off
  Switch1 : Switch  Criteria=u2 > Threshold  SaturateOnIntegerOverflow=off  InputSameDT=off
  Out1 : Outport
  wires:
  In1/1 -> Switch1/3, IsNaN1/1
  Switch1/1 -> Out1/1, Delay/1
  Delay/1 -> Switch1/1
  IsNaN1/1 -> Switch1/2

== system Quadcopter_ControllerWithNavigation/Navigation/Quadcopter Navigation Algorithm/Read waypoint from QGroundControl Mission/Guidance Subsystem/IDLE ==
  Current Position : Inport
  Action Port : ActionPort  InitializeStates=reset  ActionPortLabel=else
  Maintain Current Yaw during IDLE : Subsystem
  Mux : Mux  Inputs=2
  Reshape1 : Reshape  OutputDimensionality=Row vector (2-D)
  Selector : Selector  InputPortWidth=4  IndexOptions=Index vector (dialog)  Indices=[4]  OutputSizes=1
  Selector1 : Selector  InputPortWidth=4  IndexOptions=Index vector (dialog)  Indices=[1 2 3]  OutputSizes=1
  x_y_z_yaw : Outport
  wires:
  Maintain Current Yaw during IDLE/1(yaw_Out) -> Mux/2
  Current Position/1 -> Selector/1, Selector1/1
  Selector/1 -> Maintain Current Yaw during IDLE/1(yaw_In)
  Selector1/1 -> Mux/1
  Mux/1 -> Reshape1/1
  Reshape1/1 -> x_y_z_yaw/1

== system Quadcopter_ControllerWithNavigation/Navigation/Quadcopter Navigation Algorithm/Read waypoint from QGroundControl Mission/Guidance Subsystem/Land ==
  Current Position : Inport
  Current WP : Inport  Port=2
  Previous Waypoints : Inport  Port=3
  Action Port : ActionPort  InitializeStates=reset  ActionPortLabel=elseif(u1 ==4)
  Delay : Delay  DelayLength=1
  Ensure Smooth descend during Land : Subsystem
  IsNaN : RelationalOperator  Operator=isNaN  OutDataTypeStr=boolean  RndMeth=Simplest  InputSameDT=off
  Maintain Current Yaw during Land : Subsystem
  Mux : Mux  Inputs=3
  OR : Logic  Operator=OR  Inputs=1  IconShape=distinctive  AllPortsSameDT=off  OutDataTypeStr=boolean
  Reshape : Reshape  OutputDimensionality=Row vector (2-D)
  Reshape1 : Reshape  OutputDimensionality=Row vector (2-D)
  Selector : Selector  InputPortWidth=4  IndexOptions=Index vector (dialog)  Indices=[4]  OutputSizes=1
  Selector1 : Selector  InputPortWidth=3  IndexOptions=Index vector (dialog)  Indices=[1 2]  OutputSizes=1
  Selector2 : Selector  InputPortWidth=4  IndexOptions=Index vector (dialog)  Indices=[1 2]  OutputSizes=1
  Switch : Switch  Criteria=u2 > Threshold  SaturateOnIntegerOverflow=off  InputSameDT=off
  x_y_z_yaw : Outport
  wires:
  Delay/1 -> Switch/1
  Reshape1/1 -> Delay/1
  OR/1 -> Switch/2
  Mux/1 -> Reshape/1
  Selector1/1 -> Switch/3, IsNaN/1
  Reshape/1 -> x_y_z_yaw/1
  Current Position/1 -> Selector2/1, Selector/1
  IsNaN/1 -> OR/1
  Selector2/1 -> Reshape1/1
  Current WP/1 -> Ensure Smooth descend during Land/2(Current WP), Selector1/1
  Ensure Smooth descend during Land/1(z) -> Mux/2
  Switch/1 -> Mux/1
  Previous Waypoints/1 -> Ensure Smooth descend during Land/1(Previous Waypoints)
  Maintain Current Yaw during Land/1(yaw_Out) -> Mux/3
  Selector/1 -> Maintain Current Yaw during Land/1(yaw_In)

== system Quadcopter_ControllerWithNavigation/Navigation/Quadcopter Navigation Algorithm/Read waypoint from QGroundControl Mission/Guidance Subsystem/Take-off ==
  Current Position : Inport
  Current WP : Inport  Port=2
  Action Port : ActionPort  InitializeStates=reset  ActionPortLabel=if((u1 ==3))
  Demux : Demux
  Demux1 : Demux  Outputs=3
  Ensure smooth ascend during Takeoff : Subsystem
  Maintain Current Yaw during TakeOff : Subsystem
  Mux : Mux
  Reshape : Reshape  OutputDimensionality=Row vector (2-D)
  Terminator1 : Terminator
  Terminator2 : Terminator
  Terminator3 : Terminator
  x_y_z_yaw : Outport
  wires:
  Current Position/1 -> Demux/1
  Mux/1 -> Reshape/1
  Current WP/1 -> Demux1/1
  Demux1/3 -> Ensure smooth ascend during Takeoff/1(In1)
  Demux/3 -> Terminator3/1
  Demux/1 -> Terminator1/1
  Demux/2 -> Terminator2/1
  Demux1/1 -> Mux/1
  Demux1/2 -> Mux/2
  Reshape/1 -> x_y_z_yaw/1
  Demux/4 -> Maintain Current Yaw during TakeOff/1(yaw_In)
  Maintain Current Yaw during TakeOff/1(yaw_Out) -> Mux/4
  Ensure smooth ascend during Takeoff/1(Out1) -> Mux/3

== system Quadcopter_ControllerWithNavigation/Navigation/Quadcopter Navigation Algorithm/Read waypoint from QGroundControl Mission/Guidance Subsystem/Waypoint ==
  Current Position : Inport
  Previous Waypoints : Inport  Port=2
  Current Waypoints : Inport  Port=3
  Next Waypoints : Inport  Port=4
  Waypoint Type : Inport  Port=5
  Action Port : ActionPort  InitializeStates=reset  ActionPortLabel=elseif( u1==0)
  Constant : Constant  Value=6
  Matrix Concatenate : Concatenate  NumInputs=3  Mode=Multidimensional array
  Output signal conditioning : Subsystem
  Reshape1 : Reshape
  Terminator : Terminator
  Terminator1 : Terminator
  UAV Waypoint Follower : uavalgslib/Waypoint Follower  UAVType=multirotor  StartFrom=first  TransitionRadiusSource=internal  TransitionRadius=2  MinLookaheadDistance=0.3  YawInput=off  ShowCrossTrackErrorOutput=off  ShowStatusOutput=off  SimulateUsing=Code generation
  x_y_z_yaw : Outport
  wires:
  Constant/1 -> UAV Waypoint Follower/3
  Matrix Concatenate/1 -> UAV Waypoint Follower/2
  UAV Waypoint Follower/2 -> Terminator/1
  Reshape1/1 -> UAV Waypoint Follower/1
  Output signal conditioning/1(xyzYaw) -> x_y_z_yaw/1
  Waypoint Type/1 -> Output signal conditioning/4(Waypoint Type)
  UAV Waypoint Follower/4 -> Terminator1/1
  UAV Waypoint Follower/1 -> Output signal conditioning/2(LookAhead Point)
  UAV Waypoint Follower/3 -> Output signal conditioning/3(Desired Yaw)
  Current Waypoints/1 -> Matrix Concatenate/2
  Current Position/1 -> Reshape1/1, Output signal conditioning/1(Current Position)
  Previous Waypoints/1 -> Matrix Concatenate/1
  Next Waypoints/1 -> Matrix Concatenate/3

== system Quadcopter_ControllerWithNavigation/Navigation/Quadcopter Navigation Algorithm/Path Correction from Onboard Computer/Guidance Subsystem/IDLE/Maintain Current Yaw during IDLE ==
  yaw_In : Inport
  Constant : Constant  Value=0
  Delay : Delay  DelayLength=1  InitialCondition=1
  Enabled Subsystem2 : Subsystem  TreatAsAtomicUnit=on
  yaw_Out : Outport
  wires:
  Delay/1 -> Enabled Subsystem2/Enable
  Constant/1 -> Delay/1
  yaw_In/1 -> Enabled Subsystem2/1(yaw_In)
  Enabled Subsystem2/1(yaw_Out) -> yaw_Out/1

== system Quadcopter_ControllerWithNavigation/Navigation/Quadcopter Navigation Algorithm/Path Correction from Onboard Computer/Guidance Subsystem/Land/Ensure Smooth descend during Land ==
  note: This ensures that the landing process is smooth by continously decrementing the altitude, instead of a sudden fall.
  note: This logic takes care of the case when Land waypoint altitude is not 0
  Previous Waypoints : Inport
  Current WP : Inport  Port=2
  Delay : Delay  DelayLength=1
  Enabled Subsystem : Subsystem  TreatAsAtomicUnit=on
  Gain : Gain  Gain=-1
  Gain1 : Gain  Gain=-1
  Gain2 : Gain  Gain=-1
  GreaterThan : RelationalOperator  Operator=>  OutDataTypeStr=boolean  RndMeth=Simplest  InputSameDT=off
  Rate of descent : Constant  Value=0.02
  Selector : Selector  InputPortWidth=3  IndexOptions=Index vector (dialog)  Indices=[3]  OutputSizes=1
  Selector1 : Selector  InputPortWidth=3  IndexOptions=Index vector (dialog)  Indices=[3]  OutputSizes=1
  Subtract : Sum  Inputs=+-
  Switch : Switch  Criteria=u2 > Threshold  SaturateOnIntegerOverflow=off  InputSameDT=off
  Switch1 : Switch  Criteria=u2 > Threshold  SaturateOnIntegerOverflow=off  InputSameDT=off
  z : Outport
  wires:
  Selector/1 -> Gain/1
  Enabled Subsystem/1(Out) -> Delay/1
  Delay/1 -> Switch/1, Switch/2
  Gain/1 -> Switch/3
  Rate of descent/1 -> Subtract/2
  Subtract/1 -> Switch1/3, GreaterThan/2, Enabled Subsystem/1(In), Enabled Subsystem/Enable
  Switch/1 -> Subtract/1
  Previous Waypoints/1 -> Selector/1
  Current WP/1 -> Selector1/1
  Selector1/1 -> Gain2/1
  Gain2/1 -> Switch1/1, GreaterThan/1
  GreaterThan/1 -> Switch1/2
  Gain1/1 -> z/1
  Switch1/1 -> Gain1/1

== system Quadcopter_ControllerWithNavigation/Navigation/Quadcopter Navigation Algorithm/Path Correction from Onboard Computer/Guidance Subsystem/Land/Maintain Current Yaw during Land ==
  yaw_In : Inport
  Constant : Constant  Value=0
  Delay : Delay  DelayLength=1  InitialCondition=1
  Enabled Subsystem2 : Subsystem  TreatAsAtomicUnit=on
  yaw_Out : Outport
  wires:
  Delay/1 -> Enabled Subsystem2/Enable
  Constant/1 -> Delay/1
  yaw_In/1 -> Enabled Subsystem2/1(yaw_In)
  Enabled Subsystem2/1(yaw_Out) -> yaw_Out/1

== system Quadcopter_ControllerWithNavigation/Navigation/Quadcopter Navigation Algorithm/Path Correction from Onboard Computer/Guidance Subsystem/Take-off/Ensure smooth ascend during Takeoff ==
  In1 : Inport
  Delay : Delay  DelayLength=1
  Gain : Gain  Gain=-1
  Gain1 : Gain  Gain=-1
  Rate : Constant  Value=0.01
  Relational Operator : RelationalOperator  Operator=<=  OutDataTypeStr=boolean  RndMeth=Simplest  InputSameDT=off
  Sum : Sum  Inputs=|++
  Switch : Switch  Criteria=u2 > Threshold  SaturateOnIntegerOverflow=off  InputSameDT=off
  Out1 : Outport
  wires:
  Rate/1 -> Sum/1
  Gain/1 -> Out1/1
  Relational Operator/1 -> Switch/2
  Switch/1 -> Gain/1
  In1/1 -> Gain1/1
  Sum/1 -> Relational Operator/2, Switch/3, Delay/1
  Gain1/1 -> Switch/1, Relational Operator/1
  Delay/1 -> Sum/2

== system Quadcopter_ControllerWithNavigation/Navigation/Quadcopter Navigation Algorithm/Path Correction from Onboard Computer/Guidance Subsystem/Take-off/Maintain Current Yaw during TakeOff ==
  yaw_In : Inport
  Constant : Constant  Value=0
  Delay : Delay  DelayLength=1  InitialCondition=1
  Enabled Subsystem2 : Subsystem  TreatAsAtomicUnit=on
  yaw_Out : Outport
  wires:
  Constant/1 -> Delay/1
  Delay/1 -> Enabled Subsystem2/Enable
  Enabled Subsystem2/1(yaw_Out) -> yaw_Out/1
  yaw_In/1 -> Enabled Subsystem2/1(yaw_In)

== system Quadcopter_ControllerWithNavigation/Navigation/Quadcopter Navigation Algorithm/Path Correction from Onboard Computer/Guidance Subsystem/Waypoint/Output signal conditioning ==
  Current Position : Inport
  LookAhead Point : Inport  Port=2
  Desired Yaw : Inport  Port=3
  Waypoint Type : Inport  Port=4
  Compare To Constant : simulink/Logic and Bit Operations/Compare To Constant  relop===  const=5  OutDataTypeStr=boolean
  Constant : Constant  Value=0  SampleTime=-1
  IsNaN : RelationalOperator  Operator=isNaN  OutDataTypeStr=boolean  RndMeth=Simplest  InputSameDT=off
  IsNaN1 : RelationalOperator  Operator=isNaN  OutDataTypeStr=boolean  RndMeth=Simplest  InputSameDT=off
  Matrix Concatenate1 : Concatenate  Mode=Multidimensional array  ConcatenateDimension=2
  OR : Logic  Operator=OR  IconShape=distinctive  AllPortsSameDT=off  OutDataTypeStr=boolean
  OR1 : Logic  Operator=OR  Inputs=1  IconShape=distinctive  AllPortsSameDT=off  OutDataTypeStr=boolean
  Reshape2 : Reshape  OutputDimensionality=Row vector (2-D)
  Reshape3 : Reshape  OutputDimensionality=Row vector (2-D)
  Switch : Switch  Criteria=u2 ~= 0  SaturateOnIntegerOverflow=off  InputSameDT=off
  Switch1 : Switch  Criteria=u2 > Threshold  SaturateOnIntegerOverflow=off  InputSameDT=off
  Transpose1 : Math  Operator=transpose
  xyzYaw : Outport
  wires:
  IsNaN1/1 -> OR1/1
  Reshape2/1 -> Matrix Concatenate1/2
  Matrix Concatenate1/1 -> Switch1/3
  OR/1 -> Switch1/2
  LookAhead Point/1 -> IsNaN1/1, Transpose1/1
  Compare To Constant/1 -> OR/2
  Transpose1/1 -> Matrix Concatenate1/1
  IsNaN/1 -> Switch/2
  Reshape3/1 -> Switch1/1
  Waypoint Type/1 -> Compare To Constant/1
  Switch1/1 -> xyzYaw/1
  Current Position/1 -> Reshape3/1
  OR1/1 -> OR/1
  Constant/1 -> Switch/1
  Switch/1 -> Reshape2/1
  Desired Yaw/1 -> Switch/3, IsNaN/1

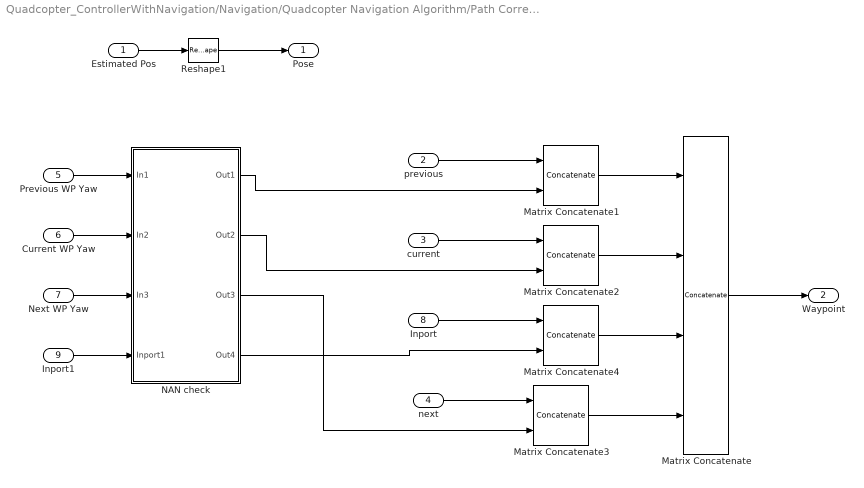
== system Quadcopter_ControllerWithNavigation/Navigation/Quadcopter Navigation Algorithm/Path Correction from Onboard Computer/Guidance Subsystem/Waypoint/Waypoints ==
  Estimated Pos : Inport
  previous : Inport  Port=2
  current : Inport  Port=3
  next : Inport  Port=4
  Previous WP Yaw : Inport  Port=5
  Current WP Yaw : Inport  Port=6
  Next WP Yaw : Inport  Port=7
  Inport : Inport  Port=8
  Inport1 : Inport  Port=9
  Matrix Concatenate : Concatenate  NumInputs=4  Mode=Multidimensional array
  Matrix Concatenate{1..4} (4 alike) : Concatenate  Mode=Multidimensional array  ConcatenateDimension=2
  NAN check : Subsystem
  Reshape1 : Reshape
  Pose : Outport
  Waypoint : Outport  Port=2
  wires:
  next/1 -> Matrix Concatenate3/1
  Matrix Concatenate/1 -> Waypoint/1
  previous/1 -> Matrix Concatenate1/1
  Estimated Pos/1 -> Reshape1/1
  Reshape1/1 -> Pose/1
  Previous WP Yaw/1 -> NAN check/1(In1)
  Current WP Yaw/1 -> NAN check/2(In2)
  Next WP Yaw/1 -> NAN check/3(In3)
  Matrix Concatenate1/1 -> Matrix Concatenate/1
  Matrix Concatenate2/1 -> Matrix Concatenate/2
  Matrix Concatenate3/1 -> Matrix Concatenate/4
  NAN check/1(Out1) -> Matrix Concatenate1/2
  NAN check/2(Out2) -> Matrix Concatenate2/2
  NAN check/3(Out3) -> Matrix Concatenate3/2
  Matrix Concatenate4/1 -> Matrix Concatenate/3
  Inport/1 -> Matrix Concatenate4/1
  Inport1/1 -> NAN check/4(Inport1)
  NAN check/4(Out4) -> Matrix Concatenate4/2
  current/1 -> Matrix Concatenate2/1

== system Quadcopter_ControllerWithNavigation/Navigation/Quadcopter Navigation Algorithm/Read waypoint from QGroundControl Mission/Guidance Subsystem/IDLE/Maintain Current Yaw during IDLE ==
  yaw_In : Inport
  Constant : Constant  Value=0
  Delay : Delay  DelayLength=1  InitialCondition=1
  Enabled Subsystem2 : Subsystem  TreatAsAtomicUnit=on
  yaw_Out : Outport
  wires:
  Delay/1 -> Enabled Subsystem2/Enable
  Constant/1 -> Delay/1
  yaw_In/1 -> Enabled Subsystem2/1(yaw_In)
  Enabled Subsystem2/1(yaw_Out) -> yaw_Out/1

== system Quadcopter_ControllerWithNavigation/Navigation/Quadcopter Navigation Algorithm/Read waypoint from QGroundControl Mission/Guidance Subsystem/Land/Ensure Smooth descend during Land ==
  note: This ensures that the landing process is smooth by continously decrementing the altitude, instead of a sudden fall.
  note: This logic takes care of the case when Land waypoint altitude is not 0
  Previous Waypoints : Inport
  Current WP : Inport  Port=2
  Delay : Delay  DelayLength=1
  Enabled Subsystem : Subsystem  TreatAsAtomicUnit=on
  Gain : Gain  Gain=-1
  Gain1 : Gain  Gain=-1
  Gain2 : Gain  Gain=-1
  GreaterThan : RelationalOperator  Operator=>  OutDataTypeStr=boolean  RndMeth=Simplest  InputSameDT=off
  Rate of descent : Constant  Value=0.02
  Selector : Selector  InputPortWidth=3  IndexOptions=Index vector (dialog)  Indices=[3]  OutputSizes=1
  Selector1 : Selector  InputPortWidth=3  IndexOptions=Index vector (dialog)  Indices=[3]  OutputSizes=1
  Subtract : Sum  Inputs=+-
  Switch : Switch  Criteria=u2 > Threshold  SaturateOnIntegerOverflow=off  InputSameDT=off
  Switch1 : Switch  Criteria=u2 > Threshold  SaturateOnIntegerOverflow=off  InputSameDT=off
  z : Outport
  wires:
  Selector/1 -> Gain/1
  Enabled Subsystem/1(Out) -> Delay/1
  Delay/1 -> Switch/1, Switch/2
  Gain/1 -> Switch/3
  Rate of descent/1 -> Subtract/2
  Subtract/1 -> Switch1/3, GreaterThan/2, Enabled Subsystem/1(In), Enabled Subsystem/Enable
  Switch/1 -> Subtract/1
  Previous Waypoints/1 -> Selector/1
  Current WP/1 -> Selector1/1
  Selector1/1 -> Gain2/1
  Gain2/1 -> Switch1/1, GreaterThan/1
  GreaterThan/1 -> Switch1/2
  Gain1/1 -> z/1
  Switch1/1 -> Gain1/1

== system Quadcopter_ControllerWithNavigation/Navigation/Quadcopter Navigation Algorithm/Read waypoint from QGroundControl Mission/Guidance Subsystem/Land/Maintain Current Yaw during Land ==
  yaw_In : Inport
  Constant : Constant  Value=0
  Delay : Delay  DelayLength=1  InitialCondition=1
  Enabled Subsystem2 : Subsystem  TreatAsAtomicUnit=on
  yaw_Out : Outport
  wires:
  Delay/1 -> Enabled Subsystem2/Enable
  Constant/1 -> Delay/1
  yaw_In/1 -> Enabled Subsystem2/1(yaw_In)
  Enabled Subsystem2/1(yaw_Out) -> yaw_Out/1
